simulink model "estimation_simu"  (R2023a)
settings: Solver=VariableStepAuto  StartTime=0.0  StopTime=Tf*n  RelTol=1e-3
values from neighbouring files (symbols this model uses):
  n = 200    [main.m]
  Tf = 3600    [main.m]
  Vo = 4.2    [main.m]
libraries: nesl_utility x7, fl_lib x7, simulink x1
settings Model: Creator=dmm  LastModifiedBy=dmm
settings OptimizationCC: ReuseModelBlockBuffer=off

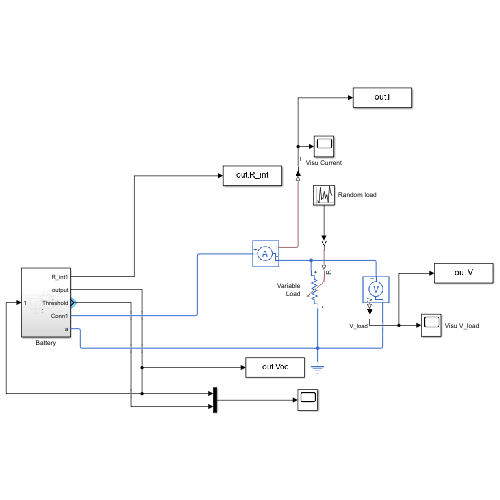
[thumbnail: Simulink's stored preview of the top-level diagram]
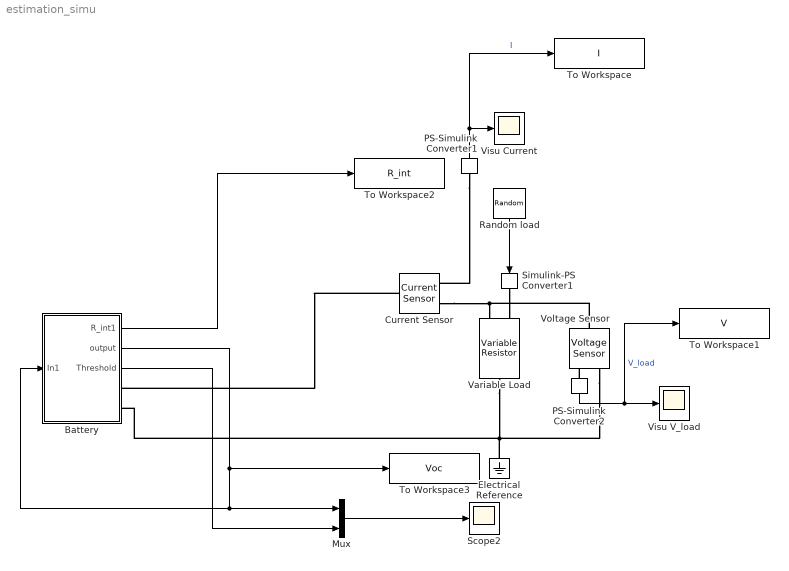
== system estimation_simu ==
  Battery : Subsystem
  Current Sensor : fl_lib/Electrical/Electrical Sensors/Current Sensor
  Electrical Reference : fl_lib/Electrical/Electrical Elements/Electrical Reference
  Mux : Mux  Inputs=2
  PS-Simulink Converter1 : nesl_utility/PS-Simulink Converter  PhysicalDomain=network_engine_domain  SubClassName=ps_output  LeftPortType=input  RightPortType=output  PseudoPeriodic=off  Frequencies=[]  VectorFormat=inherit  Unit=inherit  AffineConversion=off
  PS-Simulink Converter2 : nesl_utility/PS-Simulink Converter  PhysicalDomain=network_engine_domain  SubClassName=ps_output  LeftPortType=input  RightPortType=output  PseudoPeriodic=off  Frequencies=[]  VectorFormat=inherit  Unit=inherit  AffineConversion=off
  Random load : UniformRandomNumber  Minimum=3  Maximum=5  Seed=randi(100)  SampleTime=0.1
  Scope2 : Scope
  Simulink-PS Converter1 : nesl_utility/Simulink-PS Converter  PhysicalDomain=network_engine_domain  SubClassName=ps_input  LeftPortType=input  RightPortType=output  PseudoPeriodic=off  Frequencies=[]  NoiseDistribution=none  NoiseParameters=[]  Unit=1  AffineConversion=off  FilteringAndDerivatives=provide  SimscapeFilterOrder=1  InputFilterTimeConstant=0.001  UdotUserProvided=0
  To Workspace : ToWorkspace  VariableName=I  SaveFormat=Structure With Time  SampleTime=-1
  To Workspace1 : ToWorkspace  VariableName=V  SaveFormat=Structure With Time  SampleTime=-1
  To Workspace2 : ToWorkspace  VariableName=R_int  SaveFormat=Structure With Time  SampleTime=-1
  To Workspace3 : ToWorkspace  VariableName=Voc  SaveFormat=Structure With Time  SampleTime=-1
  Variable Load : fl_lib/Electrical/Electrical Elements/Variable Resistor  Rmin=0 Ohm  i_specify=off  i_priority=None  i=0 A  i_nominal_specify=off  i_nominal_unit=A  i_nominal_value=1  v_specify=off  v_priority=None  v=0 V  v_nominal_specify=off  v_nominal_unit=V  v_nominal_value=1
  Visu Current : Scope
  Visu V_load : Scope
  Voltage Sensor : fl_lib/Electrical/Electrical Sensors/Voltage Sensor
  wires:
  Random load/1 -> Simulink-PS Converter1/1
  PS-Simulink Converter2/1 -> To Workspace1/1, Visu V_load/1  "V_load"
  PS-Simulink Converter1/1 -> To Workspace/1, Visu Current/1  "I"
  Mux/1 -> Scope2/1
  Battery/2(output) -> To Workspace3/1, Battery/1(In1), Mux/1
  Battery/1(R_int1) -> To Workspace2/1
  Battery/3(Threshold) -> Mux/2
  connections:
  Simulink-PS Converter1/RConn1 -- Variable Load/LConn1
  Current Sensor/RConn2 -- Voltage Sensor/LConn1 -- Variable Load/LConn2
  PS-Simulink Converter1/LConn1 -- Current Sensor/RConn1
  PS-Simulink Converter2/LConn1 -- Voltage Sensor/RConn1
  Voltage Sensor/RConn2 -- Variable Load/RConn1 -- Battery/RConn2 -- Electrical Reference/LConn1
  Current Sensor/LConn1 -- Battery/RConn1

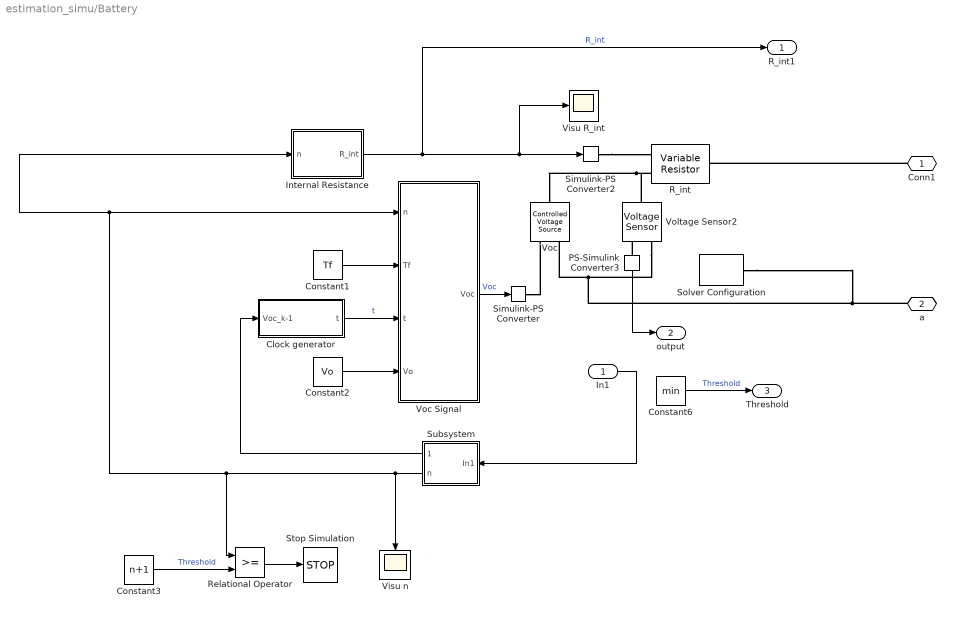
== system estimation_simu/Battery ==
  In1 : Inport
  Clock generator : Subsystem
  Constant1 : Constant  Value=Tf
  Constant2 : Constant  Value=Vo
  Constant3 : Constant  Value=n+1
  Constant6 : Constant  Value=min
  Internal Resistance : MATLAB Function  TreatAsAtomicUnit=on
  PS-Simulink Converter3 : nesl_utility/PS-Simulink Converter  PhysicalDomain=network_engine_domain  SubClassName=ps_output  LeftPortType=input  RightPortType=output  PseudoPeriodic=off  Frequencies=[]  VectorFormat=inherit  Unit=inherit  AffineConversion=off
  R_int : fl_lib/Electrical/Electrical Elements/Variable Resistor  Rmin=0 Ohm  i_specify=off  i_priority=None  i=0 A  i_nominal_specify=off  i_nominal_unit=A  i_nominal_value=1  v_specify=off  v_priority=None  v=0 V  v_nominal_specify=off  v_nominal_unit=V  v_nominal_value=1
  Relational Operator : RelationalOperator  OutDataTypeStr=boolean  RndMeth=Simplest  InputSameDT=off
  Simulink-PS Converter : nesl_utility/Simulink-PS Converter  PhysicalDomain=network_engine_domain  SubClassName=ps_input  LeftPortType=input  RightPortType=output  PseudoPeriodic=off  Frequencies=[]  NoiseDistribution=none  NoiseParameters=[]  Unit=1  AffineConversion=off  FilteringAndDerivatives=provide  SimscapeFilterOrder=1  InputFilterTimeConstant=0.001  UdotUserProvided=0
  Simulink-PS Converter2 : nesl_utility/Simulink-PS Converter  PhysicalDomain=network_engine_domain  SubClassName=ps_input  LeftPortType=input  RightPortType=output  PseudoPeriodic=off  Frequencies=[]  NoiseDistribution=none  NoiseParameters=[]  Unit=1  AffineConversion=off  FilteringAndDerivatives=provide  SimscapeFilterOrder=1  InputFilterTimeConstant=0.001  UdotUserProvided=0
  Solver Configuration : nesl_utility/Solver Configuration  PhysicalDomain=network_engine_domain  SubClassName=solver  LeftPortType=input  RightPortType=generic  Tones=[]  Harmonics=[]  SimulateNoise=off  Profile=off  UseLocalSampling=off  EnableSwitchedLinearOptims=on  FrequencyDomain=off  UseCCode=off  RelTol=0.001  AbsTol=0.001  MinStep=1e-09  ToWorkspace=off  RevertToSquareIcSolve=off  NumHomotopyIterations=100  PhasorMode=off  PhasorModeNumHarmonics=1  ConsistencySolver=NEWTON_XTOL_AFTER_FTOL  IndexReductionMethod=DerivativeReplacement  DoDC=off  ResidualTolerance=1e-09  ConsistencyTolSource=GLOBAL  ConsistencyAbsTol=0.001  ConsistencyRelTol=0.001  ConsistencyTolFactor=0.001  UseLocalSolver=off  LocalSolverChoice=NE_BACKWARD_EULER_ADVANCER  ResolveIndetEquations=on  FunctionEvalNumThread=1  LocalSolverSampleTime=0.001  DoFixedCost=off  MaxNonlinIter=3  MaxModeIter=2  ComputeImpulses=off  ImpulseIterations=2  LinearAlgebra=auto  LinearAlgebraNumThread=0  EquationFormulation=NE_TIME_EF  DelaysMemoryBudget=1024  AutomaticFiltering=on  FilteringTimeConstant=0.001  PartitionStorageMethod=AS_NEEDED  PartitionMemoryBudget=1024  PartitionMethod=ROBUST
  Stop Simulation : Stop
  Subsystem : Subsystem
  Visu R_int : Scope
  Visu n : Scope
  Voc : fl_lib/Electrical/Electrical Sources/Controlled Voltage Source
  Voc Signal : MATLAB Function  TreatAsAtomicUnit=on
  Voltage Sensor2 : fl_lib/Electrical/Electrical Sensors/Voltage Sensor
  Conn1 : PMIOPort  Side=Right
  a : PMIOPort  Port=2  Side=Right
  R_int1 : Outport
  output : Outport  Port=2
  Threshold : Outport  Port=3
  wires:
  Constant6/1 -> Threshold/1  "Threshold"
  Internal Resistance/1(R_int) -> R_int1/1, Visu R_int/1, Simulink-PS Converter2/1  "R_int"
  PS-Simulink Converter3/1 -> output/1
  Constant2/1 -> Voc Signal/4(Vo)
  Constant1/1 -> Voc Signal/2(Tf)
  Subsystem/2(n) -> Visu n/1, Relational Operator/1, Internal Resistance/1(n), Voc Signal/1(n)
  Relational Operator/1 -> Stop Simulation/1
  Constant3/1 -> Relational Operator/2  "Threshold"
  Voc Signal/1(Voc) -> Simulink-PS Converter/1  "Voc"
  Clock generator/1(t) -> Voc Signal/3(t)  "t"
  Subsystem/1(Voc_k-1) -> Clock generator/1(Voc_k-1)
  In1/1 -> Subsystem/1(In1)
  connections:
  a/RConn1 -- Solver Configuration/RConn1 -- Voltage Sensor2/RConn2 -- Voc/RConn2
  R_int/LConn2 -- Voltage Sensor2/LConn1 -- Voc/LConn1
  Simulink-PS Converter/RConn1 -- Voc/RConn1
  PS-Simulink Converter3/LConn1 -- Voltage Sensor2/RConn1
  Simulink-PS Converter2/RConn1 -- R_int/LConn1
  Conn1/RConn1 -- R_int/RConn1

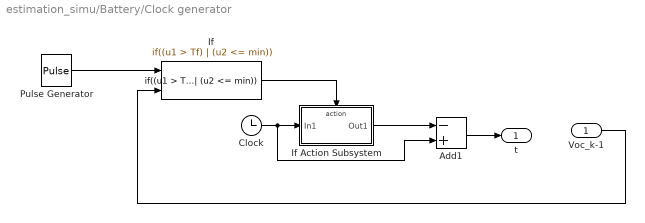
== system estimation_simu/Battery/Clock generator ==
  Voc_k-1 : Inport
  Add1 : Sum  Inputs=-+
  Clock : Clock
  If : If  NumInputs=2  IfExpression=(u1 > Tf) | (u2 <= min)  ShowElse=off
  If Action Subsystem : Subsystem  TreatAsAtomicUnit=on
  Pulse Generator : DiscretePulseGenerator  PulseType=Time based  Period=Tf  PulseWidth=5
  t : Outport
  wires:
  Voc_k-1/1 -> If/2
  Clock/1 -> Add1/2, If Action Subsystem/1(In1)
  Pulse Generator/1 -> If/1
  If/1 -> If Action Subsystem/Action
  If Action Subsystem/1(Out1) -> Add1/1
  Add1/1 -> t/1

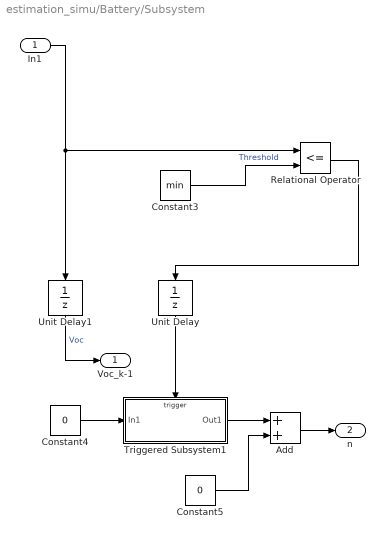
== system estimation_simu/Battery/Subsystem ==
  In1 : Inport
  Add : Sum
  Constant3 : Constant  Value=min
  Constant4 : Constant  Value=0
  Constant5 : Constant  Value=0
  Relational Operator : RelationalOperator  Operator=<=  OutDataTypeStr=boolean  RndMeth=Simplest  InputSameDT=off
  Triggered Subsystem1 : Subsystem  TreatAsAtomicUnit=on
  Unit Delay : UnitDelay  SampleTime=-1  HasFrameUpgradeWarning=on
  Unit Delay1 : UnitDelay  SampleTime=-1  HasFrameUpgradeWarning=on
  Voc_k-1 : Outport
  n : Outport  Port=2
  wires:
  Relational Operator/1 -> Unit Delay/1
  Unit Delay/1 -> Triggered Subsystem1/Trigger
  Constant3/1 -> Relational Operator/2  "Threshold"
  Triggered Subsystem1/1(Out1) -> Add/1
  Constant5/1 -> Add/2
  In1/1 -> Unit Delay1/1, Relational Operator/1
  Constant4/1 -> Triggered Subsystem1/1(In1)
  Add/1 -> n/1
  Unit Delay1/1 -> Voc_k-1/1  "Voc"

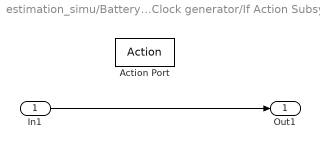
== system estimation_simu/Battery/Clock generator/If Action Subsystem ==
  In1 : Inport
  Action Port : ActionPort  ActionPortLabel=if((u1 > Tf) | (u2 <= min))
  Out1 : Outport
  wires:
  In1/1 -> Out1/1

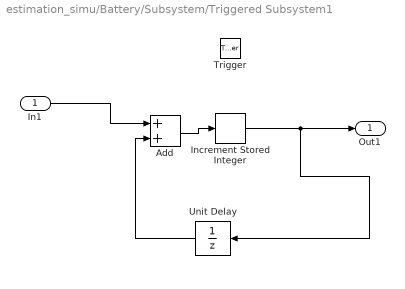
== system estimation_simu/Battery/Subsystem/Triggered Subsystem1 ==
  In1 : Inport  OutDataTypeStr=double  LockScale=on
  Trigger : TriggerPort  VariantControl=(inherit)
  Add : Sum
  Increment Stored Integer : simulink/Additional Math & Discrete/Additional Math: Increment - Decrement/Increment Stored Integer
  Unit Delay : UnitDelay  SampleTime=-1  HasFrameUpgradeWarning=on
  Out1 : Outport
  wires:
  Increment Stored Integer/1 -> Out1/1, Unit Delay/1
  In1/1 -> Add/1
  Add/1 -> Increment Stored Integer/1
  Unit Delay/1 -> Add/2

== matlab function estimation_simu/Battery/Voc Signal ==
  data: n input; Voc output; Tf input; t input; Vo input
function Voc = fcn(n, Tf, t, Vo)
    
    b = (tan(1.5)/1.8) - ((tan(-((3503.67-11.17*n)/(Tf-9.87*n)) + 1.5))/1.8);
    a = Vo  - tan(1.5)/b;
    c = pi/(Tf-9.87*n);

    Voc = a + tan(-t*c + 1.5)/b;

end

== matlab function estimation_simu/Battery/Internal Resistance ==
  data: n input; R_int output
function R_int = fcn(n)
    R_int = 0.06 + 8.4375E-5*n;
end
